simulink model "MalhaFechada"  (R2024a)
settings: Solver=VariableStepAuto  StartTime=0.0  StopTime=10.0  RelTol=1e-3
undefined symbols (not defined in the file): K
settings Model: Creator=ottoc  LastModifiedBy=acram
settings SolverCC: AlgebraicLoopSolver=TrustRegion
settings DataIOCC: ReturnWorkspaceOutputs=off
settings DebuggingCC: UnconnectedInputMsg=warning  UnconnectedOutputMsg=warning  UnconnectedLineMsg=warning  ArithmeticOperatorsInVariantConditions=warning
settings ModelReferenceCC: EnableRefExpFcnMdlSchedulingChecks=on
settings SFSimCC: CustomCodeUndefinedFunction=UseInterfaceOnly
settings RTWCC: GPUComputeCapability=3.5

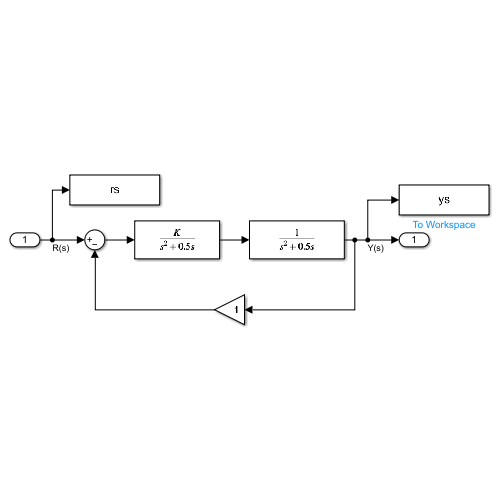
[thumbnail: Simulink's stored preview of the top-level diagram]
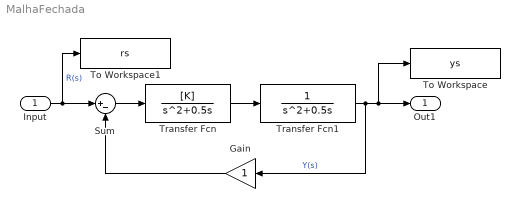
== system MalhaFechada ==
  Input : Inport
  Gain : Gain
  Sum : Sum  Inputs=|+-
  To Workspace : ToWorkspace  VariableName=ys  SaveFormat=Structure With Time  SampleTime=-1
  To Workspace1 : ToWorkspace  VariableName=rs  SaveFormat=Structure With Time  SampleTime=-1
  Transfer Fcn : TransferFcn  Numerator=[K]  Denominator=[1 0.5 0]
  Transfer Fcn1 : TransferFcn  Denominator=[1 0.5 0]
  Out1 : Outport  VectorParamsAs1DForOutWhenUnconnected=off
  wires:
  Sum/1 -> Transfer Fcn/1
  Transfer Fcn/1 -> Transfer Fcn1/1
  Transfer Fcn1/1 -> To Workspace/1, Out1/1, Gain/1  "Y(s)"
  Gain/1 -> Sum/2
  Input/1 -> To Workspace1/1, Sum/1  "R(s)"
